simulink model "mpc_test"  (R2015a)
settings: Solver=ode45  StartTime=0.0  StopTime=200  RelTol=1e-3
libraries: cstblocks x1, mpclib x1, dspsrcs4 x1
settings Model: Creator=Szymon  LastModifiedBy=Szymon

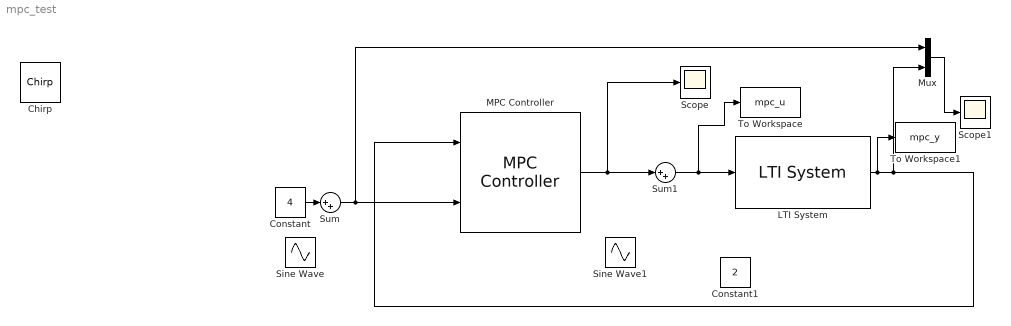
== system mpc_test ==
  Constant : Constant  Value=4
  Constant1 : Constant  Value=2
  LTI System : cstblocks/LTI System  sys=inertiaStateSpace  IC=[]
  MPC Controller : mpclib/MPC Controller  SCDEnableBlockLinearizationSpecification=on  mpcobj=MPCobj  is_multiple=0  enable_value=0  n_mv=1  n_mo=1  n_md=0  n_ts=0.1  is_designfromscratch=0  return_u0=off  ref_from_ws=off  ref_signal_name=[]  ref_preview=off  md_from_ws=off  md_signal_name=[]  md_preview=off  from_project=off  project_file=MPCtask.mat  md_inport=off  mv_inport=off  cost_outport=off  return_sequence=off  return_qpstatus=off  return_state=off  state_inport=off  lims_inport=off  ywt_inport=off  uwt_inport=off  duwt_inport=off  rhoeps_inport=off  uref_inport=off  BlockDataType=double  SampleTimeInherited=off  switch_inport=off
  Mux : Mux  Inputs=2
  Scope : Scope
  Scope1 : Scope
  Sine Wave : Sin  Amplitude=2  Frequency=0.1  SampleTime=0
  Sine Wave1 : Sin  Frequency=0.05  SampleTime=0
  Sum : Sum  Inputs=|++
  Sum1 : Sum  Inputs=|++
  To Workspace : ToWorkspace  VariableName=mpc_u  SampleTime=0.1
  To Workspace1 : ToWorkspace  VariableName=mpc_y  SampleTime=0.1
  Chirp : dspsrcs4/Chirp  IOType=siggen  sweep=Linear  mode=Unidirectional  f0=1000  f1=4000  t1=1  Tsweep=1  phase=0  Ts=1/8000  spf=1  datatype=Double
  wires:
  MPC Controller/1 -> Sum1/1, Scope/1
  LTI System/1 -> To Workspace1/1, Mux/2, MPC Controller/1
  Constant/1 -> Sum/1
  Sum/1 -> Mux/1, MPC Controller/2
  Sum1/1 -> To Workspace/1, LTI System/1
  Mux/1 -> Scope1/1
